simulink model "autoware_path_subscriber"  (R2025b)
settings: Solver=VariableStepAuto  StartTime=0.0  StopTime=10.0  RelTol=1e-3
libraries: ros2lib x2
settings Model: Creator=omer  LastModifiedBy=omer

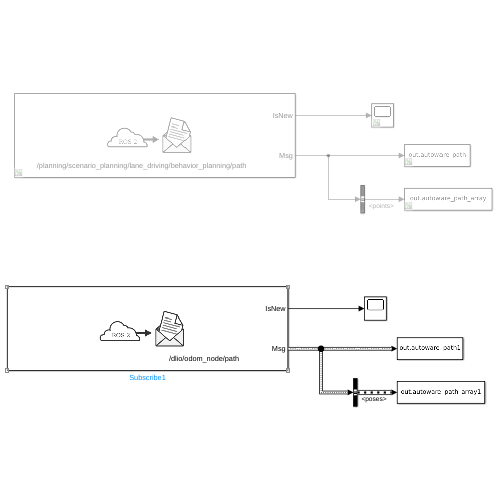
[thumbnail: Simulink's stored preview of the top-level diagram]
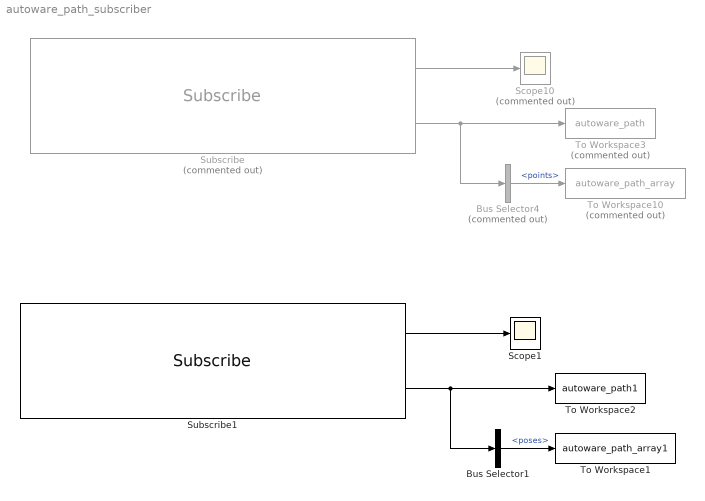
== system autoware_path_subscriber ==
  Bus Selector1 : BusSelector  OutputSignals=poses
  Bus Selector4 : BusSelector  Commented=on  OutputSignals=points
  Scope1 : Scope
      settings: ActiveDisplayYMinimum=-5.7838392804365668  ActiveDisplayYMaximum=6.0362745040519554
  Scope10 : Scope  Commented=on
      settings: ActiveDisplayYMinimum=-2.1920698371442371  ActiveDisplayYMaximum=1.9657865216785007  DataLoggingVariableName=ScopeData10
  Subscribe : ros2lib/Subscribe  Commented=on  topicSource=Select from ROS network  topic=/planning/scenario_planning/lane_driving/behavior_planning/path  messageType=autoware_planning_msgs/Path  sampleTime=-1  QOSHistory=Keep last  QOSDepth=10  QOSReliability=Reliable  QOSDurability=Volatile  QOSDeadline=Inf  QOSLifespan=Inf  QOSLiveliness=Automatic  QOSLeaseDuration=Inf  QOSAvoidROSNamespaceConventions=off
  Subscribe1 : ros2lib/Subscribe  topicSource=Select from ROS network  topic=/dlio/odom_node/path  messageType=nav_msgs/Path  sampleTime=-1  QOSHistory=Keep last  QOSDepth=10  QOSReliability=Reliable  QOSDurability=Volatile  QOSDeadline=Inf  QOSLifespan=Inf  QOSLiveliness=Automatic  QOSLeaseDuration=Inf  QOSAvoidROSNamespaceConventions=off
  To Workspace1 : ToWorkspace  VariableName=autoware_path_array1  SaveFormat=Timeseries  SampleTime=-1
      settings: Save2DSignal=2-D array (concatenate along first dimension)
  To Workspace10 : ToWorkspace  Commented=on  VariableName=autoware_path_array  SaveFormat=Timeseries  SampleTime=-1
      settings: Save2DSignal=2-D array (concatenate along first dimension)
  To Workspace2 : ToWorkspace  VariableName=autoware_path1  SaveFormat=Timeseries  SampleTime=-1
  To Workspace3 : ToWorkspace  Commented=on  VariableName=autoware_path  SaveFormat=Timeseries  SampleTime=-1
  wires:
  Subscribe/2 -> Bus Selector4/1, To Workspace3/1
  Bus Selector4/1 -> To Workspace10/1  "<points>"
  Subscribe/1 -> Scope10/1
  Subscribe1/2 -> Bus Selector1/1, To Workspace2/1
  Subscribe1/1 -> Scope1/1
  Bus Selector1/1 -> To Workspace1/1  "<poses>"
